simulink model "my_first_model"  (R2021b)
settings: Solver=VariableStepAuto  StartTime=0.0  StopTime=10.0  RelTol=1e-3
settings Model: Creator=admin  LastModifiedBy=admin

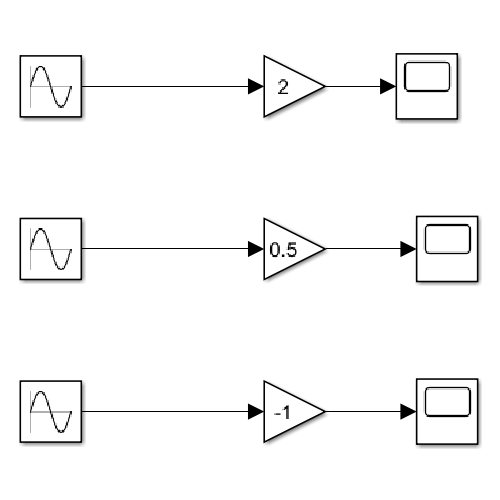
[thumbnail: Simulink's stored preview of the top-level diagram]
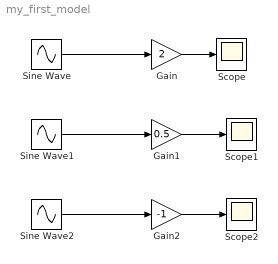
== system my_first_model ==
  Gain : Gain  Gain=2
  Gain1 : Gain  Gain=0.5
  Gain2 : Gain  Gain=-1
  Scope : Scope
  Scope1 : Scope
  Scope2 : Scope
  Sine Wave : Sin  SampleTime=0
  Sine Wave1 : Sin  SampleTime=0
  Sine Wave2 : Sin  SampleTime=0
  wires:
  Sine Wave/1 -> Gain/1
  Gain/1 -> Scope/1
  Sine Wave1/1 -> Gain1/1
  Gain1/1 -> Scope1/1
  Sine Wave2/1 -> Gain2/1
  Gain2/1 -> Scope2/1
